simulink model "bicopter_dynamics"  (R2019a)
settings: Solver=ode4  StartTime=0.0  StopTime=25  FixedStep=0.001  RelTol=1e-3
undefined symbols (not defined in the file or in its folder): Discrete, Time
libraries: ctrlSharedLib x1, simulink x1
settings Model: Creator=crsmyth  LastModifiedBy=crs20

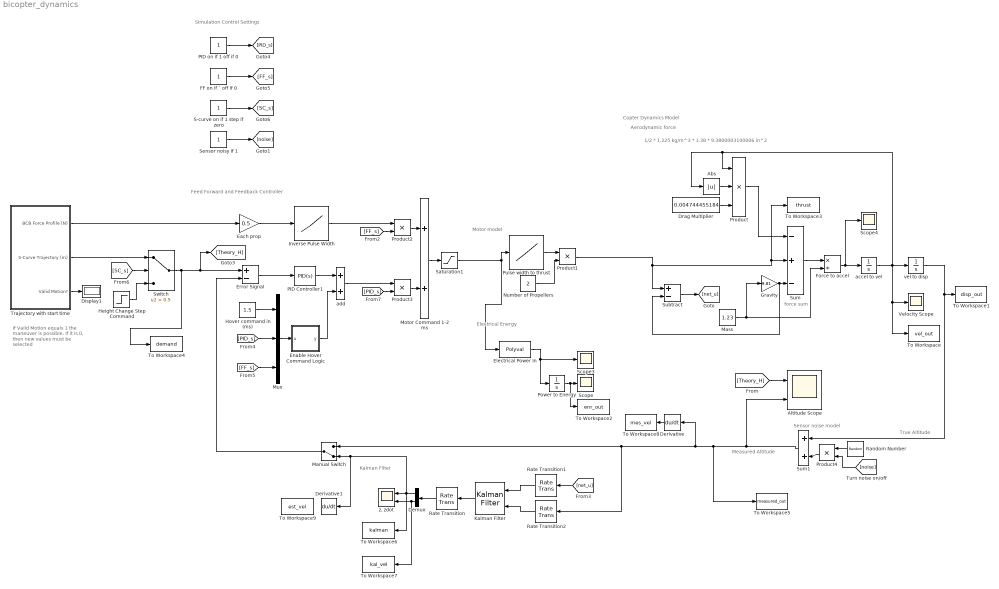
== system bicopter_dynamics ==
  note: Kalman Filter
  note: Copter Dynamics Model
  note: Measured Altitude
  note: True Altitude
  note: Sensor noise model
  note: Electrical Energy
  note: force sum
  note: Motor model
  note: Aerodynamic force
  note: 1/2 * 1.225 kg/m^3 * 1.38 * 9.3800003100006 in^2
  note: Simulation Control Settings
  note: If Valid Motion equals 1
      | the maneuver is possible.
      | If it is 0, then new values
      | must be selected
  note: Feed Forward and
      | Feedback Controller
  Abs : Abs
  Altitude Scope : Scope  NumInputPorts=2
  Demux : Demux  Outputs=2
  Derivative : Derivative
  Derivative1 : Derivative
  Display1 : Display
  Drag Multiplier : Constant  Value=0.004744455184
  Each prop : Gain  Gain=0.5
  Electrical Power In : Polyval  Coefs=[2.956191832898671e+02, -6.235353126465623e+02, 3.330393150826374e+02]
  Enable Hover Command Logic : MATLAB Function  TreatAsAtomicUnit=on
  Error Signal : Sum  Inputs=+-
  FF on if ` off if 0 : Constant
  Force to accel : Product  Inputs=*/
  Gravity : Gain  Gain=9.81
  Height Change Step Command : Step  Time=5  SampleTime=0
  Hover command in (ms) : Constant  Value=1.5
  Inverse Pulse Width : Lookup_n-D  NumberOfTableDimensions=1  BreakpointsForDimension1=[0, 9]  Table=[1, 2]  InternalRulePriority=Speed  RndMeth=Simplest  InputSameDT=on
  Kalman Filter : ctrlSharedLib/Kalman Filter  TimeDomain=Discrete-Time  UseCurrentEstimator=on  ModelSource=Individual A, B, C, D matrices  ModelSourceVariable=ss(0.95,1,1,0,1)  A=[1, 0.001; 0, 1]  B=[0.001^2 / (2 * 1.23); 0.001 / 1.23]  C=[1, 0]  D=0  NumberOfStates=1  NumberOfInputs=1  NumberOfOutputs=1  InitialEstimateSource=Dialog  X0=[0, 0]  P0=10  UseK=off  UseGH=off  NumberOfProcessNoiseInputs=1  G=1  TimeInvariantG=on  H=0  TimeInvariantH=on  Q=0.0001  TimeInvariantQ=on  R=0.01  TimeInvariantR=on  N=0  TimeInvariantN=on  AddInputPort=on  AddEnablePort=off  OutputEstimatedY=off  OutputP=off  Ts=0.001
      settings: SourceProductBaseCode=CT
  Manual Switch : ManualSwitch  CurrentSetting=0
  Mass : Constant  Value=1.23
  Motor Command 1-2 ms : Sum
  Mux : Mux  Inputs=3
  Number of Propellers : Constant  Value=2
  PID Controller1 : simulink/Continuous/PID Controller  Controller=PID  Form=Parallel  TimeDomain=Continuous-time  SampleTime=-1  IntegratorMethod=Forward Euler  FilterMethod=Forward Euler  ControllerParametersSource=internal  P=.2  I=.1  D=.1  UseFilter=on  N=10  TunerSelectOption=Transfer Function Based (PID Tuner App)  InitialConditionSource=internal  InitialConditionForIntegrator=0  InitialConditionForFilter=0  DifferentiatorICPrevScaledInput=0  ExternalReset=none  TrackingMode=off  Kt=1  LimitOutput=off  UpperSaturationLimit=inf  LowerSaturationLimit=-inf  LinearizeAsGain=on  AntiWindupMode=none  Kb=1  POutMin=[]  POutMax=[]  IOutMin=[]  IOutMax=[]  DOutMin=[]  DOutMax=[]  NOutMin=[]  NOutMax=[]  SumOutMin=[]  SumOutMax=[]  SaturationOutMin=[]  SaturationOutMax=[]  PParamMin=[]  PParamMax=[]  IParamMin=[]  IParamMax=[]  DParamMin=[]  DParamMax=[]  NParamMin=[]  NParamMax=[]  KbParamMin=[]  KbParamMax=[]  KtParamMin=[]  KtParamMax=[]  KbOutMin=[]  KbOutMax=[]  KtOutMin=[]  KtOutMax=[]  IntegratorOutMin=[]  IntegratorOutMax=[]  FilterOutMin=[]  FilterOutMax=[]  SumI1OutMin=[]  SumI1OutMax=[]  SumI2OutMin=[]  SumI2OutMax=[]  SumI3OutMin=[]  SumI3OutMax=[]  SumI4OutMin=[]  SumI4OutMax=[]  SumDOutMin=[]  SumDOutMax=[]  DifferentiatorOutMin=[]  DifferentiatorOutMax=[]  FilterDiffOutCoefMin=[]  FilterDiffOutCoefMax=[]  ReciprocalOutMin=[]  ReciprocalOutMax=[]  SumDenOutMin=[]  SumDenOutMax=[]  SumNumOutMin=[]  SumNumOutMax=[]  DivideOutMin=[]  DivideOutMax=[]  IntegratorContinuousStateAttributes=''  IntegratorStateMustResolveToSignalObject=off  IntegratorRTWStateStorageClass=Auto  FilterContinuousStateAttributes=''  FilterStateMustResolveToSignalObject=off  FilterRTWStateStorageClass=Auto  ParallelPVariant=InternalParameters  IdealPVariant=Disabled  IVariant=InternalParameters  DVariant=InternalParameters  IntegratorVariant=Continuous  SatVariant=Disabled  AWVariant=Passthrough  PCopyVariant=Disabled  TRVariant=Disabled  FdbkBlocksVariant=Forward  IdealPFdbkVariant=Disabled  SatFdbkVariant=Disabled  DerivativeFilterVariant=ContFilter  NVariant=InternalParameters  NCopyVariant=Disabled  FilterICVariant=InternalICsFilter  IntegratorICVariant=InternalICs  ExternalResetVariant=Disabled  TRSumVariant=Passthrough  SumFdbkVariant=Disabled  SumVariant=Sum_PID
  PID on if 1 off if 0 : Constant
  Power to Energy : Integrator
  Product : Product  Inputs=3
  Product{1..4} (4 alike) : Product
  Pulse width to thrust : Lookup_n-D  NumberOfTableDimensions=1  BreakpointsForDimension1=[0, 1, 2]  Table=[0, 0, 9]  InternalRulePriority=Speed  RndMeth=Simplest  InputSameDT=on
  Random Number : RandomNumber  Variance=0.01  SampleTime=0.001
  Rate Transition : RateTransition  OutPortSampleTimeOpt=Inherit
  Rate Transition1 : RateTransition  OutPortSampleTimeOpt=Inherit
  Rate Transition2 : RateTransition  OutPortSampleTimeOpt=Inherit
  S-curve on if 1 step if zero : Constant
  Saturation1 : Saturate  UpperLimit=2.0  LowerLimit=1
  Scope : Scope
  Scope3 : Scope
  Scope4 : Scope
  Sensor noisy if 1 : Constant
  Subtract : Sum  Inputs=+-
  Sum : Sum  Inputs=-+-
  Sum1 : Sum
  Switch : Switch  Criteria=u2 > Threshold  Threshold=0.5
  To Workspace : ToWorkspace  VariableName=vel_out  SaveFormat=Timeseries  SampleTime=-1
      settings: Save2DSignal=2-D array (concatenate along first dimension)
  To Workspace1 : ToWorkspace  VariableName=disp_out  SaveFormat=Timeseries  SampleTime=-1
      settings: Save2DSignal=2-D array (concatenate along first dimension)
  To Workspace2 : ToWorkspace  VariableName=enr_out  SaveFormat=Timeseries  SampleTime=-1
  To Workspace3 : ToWorkspace  VariableName=thrust  SaveFormat=Timeseries  SampleTime=-1
  To Workspace4 : ToWorkspace  VariableName=demand  SaveFormat=Timeseries  SampleTime=-1
  To Workspace5 : ToWorkspace  VariableName=measured_out  SaveFormat=Timeseries  SampleTime=-1
  To Workspace6 : ToWorkspace  VariableName=kalman  SaveFormat=Timeseries  SampleTime=-1
  To Workspace7 : ToWorkspace  VariableName=kal_vel  SaveFormat=Timeseries  SampleTime=-1
  To Workspace8 : ToWorkspace  VariableName=mes_vel  SaveFormat=Timeseries  SampleTime=-1
  To Workspace9 : ToWorkspace  VariableName=est_vel  SaveFormat=Timeseries  SampleTime=-1
  Trajectory with start time : Subsystem  mask{fA=1, dT=4, xF=1, mass=1.23, tm=0}
      mask prompts: fA "Max Force Pulse Amplitude (N)"; dT "Desired Maneuver time (sec)"; xF "Height Change (m)"; mass "Mass of Copter (kg)"; tm "Start Move Time (sec)"
  Velocity Scope : Scope
  accel to vel : Integrator
  add : Sum
  vel to disp : Integrator
  "z, zdot" : Scope  NumInputPorts=2
  wires:
  Sum/1 -> Force to accel/1
  Mass/1 -> Force to accel/2, Gravity/1
  Force to accel/1 -> Scope4/1, accel to vel/1
  Gravity/1 -> Subtract/2, Sum/3
  Product/1 -> Sum/1
  Drag Multiplier/1 -> Product/3
  Abs/1 -> Product/2
  Product1/1 -> Subtract/1, To Workspace3/1, Sum/2
  Number of Propellers/1 -> Product1/2
  Pulse width to thrust/1 -> Product1/1
  accel to vel/1 -> vel to disp/1, Abs/1, Product/1, To Workspace/1, Velocity Scope/1
  Electrical Power In/1 -> Scope3/1, Power to Energy/1
  Power to Energy/1 -> To Workspace2/1, Scope/1
  Saturation1/1 -> Pulse width to thrust/1, Electrical Power In/1
  vel to disp/1 -> Sum1/1, To Workspace1/1
  Mux/1 -> Enable Hover Command Logic/1(u)
  PID Controller1/1 -> add/1
  [SC_s] -> Switch/2
  Motor Command 1-2 ms/1 -> Saturation1/1
  Trajectory with start time/1(BCB Force Profile (N)) -> Each prop/1
  FF on if ` off if 0/1 -> [FF_s]
  [FF_s] -> Mux/3
  Enable Hover Command Logic/1(y) -> add/2
  PID on if 1 off if 0/1 -> [PID_s]
  Product2/1 -> Motor Command 1-2 ms/1
  Hover command in (ms)/1 -> Mux/1
  Product3/1 -> Motor Command 1-2 ms/2
  S-curve on if 1 step if zero/1 -> [SC_s]
  [PID_s] -> Mux/2
  [FF_s] -> Product2/2
  [PID_s] -> Product3/2
  Height Change Step Command/1 -> Switch/3
  Error Signal/1 -> PID Controller1/1
  Switch/1 -> To Workspace4/1, [Theory_H], Error Signal/1
  Trajectory with start time/2(S-Curve Trajectory (m)) -> Switch/1
  Trajectory with start time/3(Valid Motion?) -> Display1/1
  add/1 -> Product3/1
  Each prop/1 -> Inverse Pulse Width/1
  Inverse Pulse Width/1 -> Product2/1
  Sum1/1 -> Altitude Scope/2, To Workspace5/1, Derivative/1, Rate Transition2/1, Manual Switch/1
  [Theory_H] -> Altitude Scope/1
  Product4/1 -> Sum1/2
  Random Number/1 -> Product4/1
  [noise] -> Product4/2
  Sensor noisy if 1/1 -> [noise]
  Demux/1 -> "z, zdot"/1, To Workspace6/1, Derivative1/1, Manual Switch/2
  Rate Transition/1 -> Demux/1
  Kalman Filter/1 -> Rate Transition/1
  Rate Transition1/1 -> Kalman Filter/1
  Rate Transition2/1 -> Kalman Filter/2
  Subtract/1 -> [net_u]
  [net_u] -> Rate Transition1/1
  Manual Switch/1 -> Error Signal/2
  Demux/2 -> "z, zdot"/2, To Workspace7/1
  Derivative/1 -> To Workspace8/1

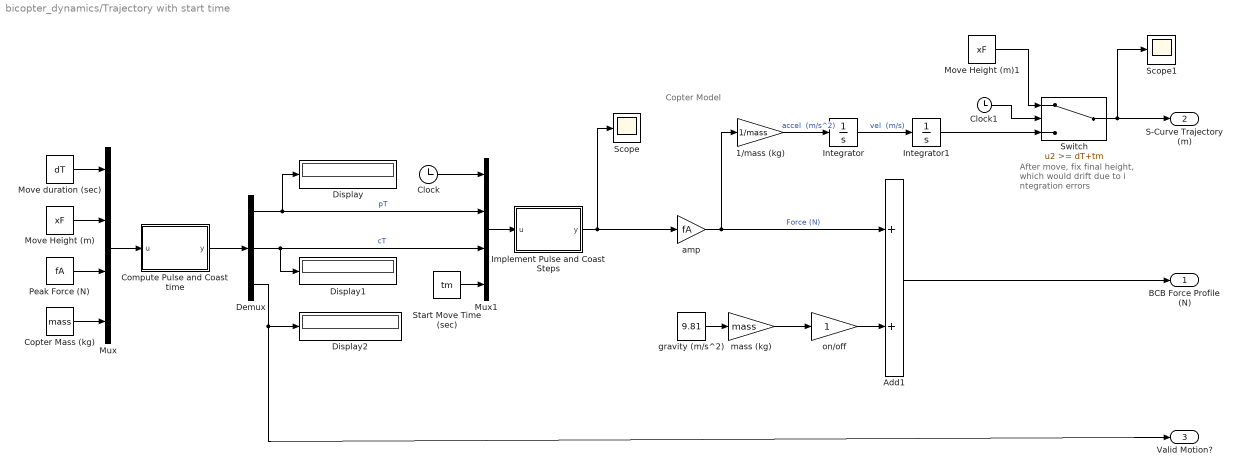
== system bicopter_dynamics/Trajectory with start time ==
  note: After move, fix final height,
      | which would drift due to i
      | ntegration errors
  note: Copter Model
  1/mass (kg) : Gain  Gain=1/mass
  Add1 : Sum
  Clock : Clock
  Clock1 : Clock
  Compute Pulse and Coast time : MATLAB Function  TreatAsAtomicUnit=on
  Copter Mass (kg) : Constant  Value=mass
  Demux : Demux  Outputs=3
  Display : Display
  Display1 : Display
  Display2 : Display
  Implement Pulse and Coast Steps : MATLAB Function  TreatAsAtomicUnit=on
  Integrator : Integrator
  Integrator1 : Integrator
  Move Height (m)1 : Constant  Value=xF
  Move Height (m) : Constant  Value=xF
  Move duration (sec) : Constant  Value=dT
  Mux : Mux
  Mux1 : Mux
  "Peak Force (N) " : Constant  Value=fA
  Scope : Scope
  Scope1 : Scope
  Start Move Time (sec) : Constant  Value=tm
  Switch : Switch  Threshold=dT+tm
  amp : Gain  Gain=fA
  gravity (m/s^2) : Constant  Value=9.81
  mass (kg) : Gain  Gain=mass
  on/off : Gain
  BCB Force Profile (N) : Outport
  S-Curve Trajectory (m) : Outport  Port=2
  Valid Motion? : Outport  Port=3
  wires:
  Add1/1 -> BCB Force Profile (N)/1
  Compute Pulse and Coast time/1(y) -> Demux/1
  Demux/1 -> Display/1, Mux1/2  "pT"
  Demux/2 -> Display1/1, Mux1/3  "cT"
  Move duration (sec)/1 -> Mux/1
  Move Height (m)/1 -> Mux/2
  "Peak Force (N) "/1 -> Mux/3
  Copter Mass (kg)/1 -> Mux/4
  Mux/1 -> Compute Pulse and Coast time/1(u)
  amp/1 -> Add1/1, 1/mass (kg)/1  "Force (N)"
  gravity (m/s^2)/1 -> mass (kg)/1
  1/mass (kg)/1 -> Integrator/1  "accel  (m/s^2)"
  mass (kg)/1 -> on/off/1
  Switch/1 -> S-Curve Trajectory (m)/1, Scope1/1
  Integrator/1 -> Integrator1/1  "vel  (m/s)"
  Clock/1 -> Mux1/1
  Mux1/1 -> Implement Pulse and Coast Steps/1(u)
  Implement Pulse and Coast Steps/1(y) -> Scope/1, amp/1
  Demux/3 -> Display2/1, Valid Motion?/1
  Clock1/1 -> Switch/2
  Integrator1/1 -> Switch/3
  Move Height (m)1/1 -> Switch/1
  Start Move Time (sec)/1 -> Mux1/4
  on/off/1 -> Add1/2

== matlab function bicopter_dynamics/Trajectory with start time/Implement Pulse and Coast Steps ==
  data: u input; y output
function y = fcn(u)
%#codegen


t  = u(1);
pT = u(2);
cT = u(3);
tm = u(4); % (sec) when to implement BCB 

if tm < 0 % error check inputs
  tm = 0;
end

if(t < tm)
  d = -1;
else
  d = 0;
end

if(t >= pT+tm)
  a = -1;
else
  a = 0;
end

if(t >= pT+cT+tm)
  b = -1;
else
  b = 0;
end

if(t >= (2*pT+cT)+tm)
  c = 1;
else
  c = 0;
end

y = 1 + a + b + c + d;

== matlab function bicopter_dynamics/Trajectory with start time/Compute Pulse and Coast time ==
  data: u input; y output
function y = fcn(u)
%#codegen

% Gordon Parker
% Michigan Technological University
% 08 Jan 2015

% Modified by Eddy Trinklein
% 27 Sept 2016


% calculates a bang-coast-bang force input to move the copter from
% rest to rest vertically. 
%
% Dialog inputs:
% dT:   desired maneuver time (sec)
% xF:   altitude change (m)
% fA:   desired force amplitude (N)
% mass: mass of copter (kg)

% Outputs:
% pTActual:  Computed pulse times (sec)
% cTActual:  coast time (sec)


dT   = u(1);
xF   = u(2);
fA   = u(3);
mass = u(4);

y = zeros(1,3);

aA = fA/mass;


tmp1 = dT^2 - 4*xF/aA;
if tmp1 < 0
  dTWorks = sqrt(4*xF/aA);
  aAWorks = 4*xF/dT^2;
  xFWorks = fA/4*dT^2;
  fprintf('This set of inputs will not work you can either:\n');
  fprintf('1) Use a maneuver time of %f\n',dTWorks);
  fprintf('2) Use a force amplitude of %f\n',aAWorks*mass);
  fprintf('3) Use a final distance of %f\n',xFWorks);
  y = [.1,.1,0];
  return;
end

%% Create Solution

% Calc pulse times that work
pT = roots([1 -dT xF/aA]); % (sec)

% pick the shortest duration pulse
pTActual = min(pT); % (sec)

% set coast time
cTActual = dT - 2*pTActual; % (sec)
  

y = [real(pTActual),real(cTActual),1];

== matlab function bicopter_dynamics/Enable Hover Command Logic ==
  data: u input; y output
function y = fcn(u)

PID = u(2);
FF  = u(3);

if ((PID > 0.5) && (FF > 0.5))
  y = 0;
elseif (PID > 0.5) && (FF < 0.5)
  y = u(1);     
elseif (PID < 0.5) && (FF > 0.5)
  y = 0;
else 
  y = 0;
end
